simulink model "Discrete_Model_Controlled"  (R2020b)
settings: Solver=VariableStepAuto  StartTime=0.0  StopTime=0.3  RelTol=1e-3
undefined symbols (not defined in the file or in its folder): C1_d, C2_d, sys_id_dec, ts
settings Model: Creator=Víctor Carmona  LastModifiedBy=Víctor Carmona
settings DataIOCC: ReturnWorkspaceOutputs=off

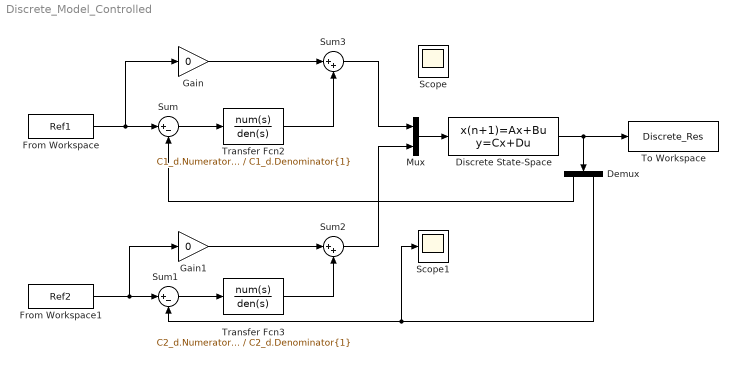
== system Discrete_Model_Controlled ==
  Demux : Demux  Outputs=2
  Discrete State-Space : DiscreteStateSpace  A=sys_id_dec.A  B=sys_id_dec.B  C=sys_id_dec.C  D=sys_id_dec.D  SampleTime=ts
  From Workspace : FromWorkspace  VariableName=Ref1  SampleTime=[ts,0]
  From Workspace1 : FromWorkspace  VariableName=Ref2  SampleTime=[ts,0]
  Gain : Gain  Gain=0
  Gain1 : Gain  Gain=0
  Mux : Mux  Inputs=2
  Scope : Scope
  Scope1 : Scope
  Sum : Sum  Inputs=|+-
  Sum1 : Sum  Inputs=|+-
  Sum2 : Sum  Inputs=|++
  Sum3 : Sum  Inputs=|++
  To Workspace : ToWorkspace  VariableName=Discrete_Res  SampleTime=ts
      settings: Save2DSignal=2-D array (concatenate along first dimension)
  Transfer Fcn2 : TransferFcn  Numerator=C1_d.Numerator{1}  Denominator=C1_d.Denominator{1}
  Transfer Fcn3 : TransferFcn  Numerator=C2_d.Numerator{1}  Denominator=C2_d.Denominator{1}
  wires:
  From Workspace/1 -> Gain/1, Sum/1
  Sum/1 -> Transfer Fcn2/1
  From Workspace1/1 -> Gain1/1, Sum1/1
  Discrete State-Space/1 -> Demux/1, To Workspace/1
  Transfer Fcn2/1 -> Sum3/2
  Gain/1 -> Sum3/1
  Sum1/1 -> Transfer Fcn3/1
  Transfer Fcn3/1 -> Sum2/2
  Gain1/1 -> Sum2/1
  Demux/1 -> Sum/2
  Demux/2 -> Scope1/1, Sum1/2
  Sum2/1 -> Mux/2
  Sum3/1 -> Mux/1
  Mux/1 -> Discrete State-Space/1
